simulink model "sampleModel2045_3_sub_sub"  (R2023a)
settings: Solver=VariableStepAuto  StartTime=0.0  StopTime=10.0  RelTol=1e-3
libraries: hdlsllib x5, simulink x2
settings Model: Creator=user1  LastModifiedBy=user1
settings OptimizationCC: BlockReduction=off  ConditionallyExecuteInputs=off

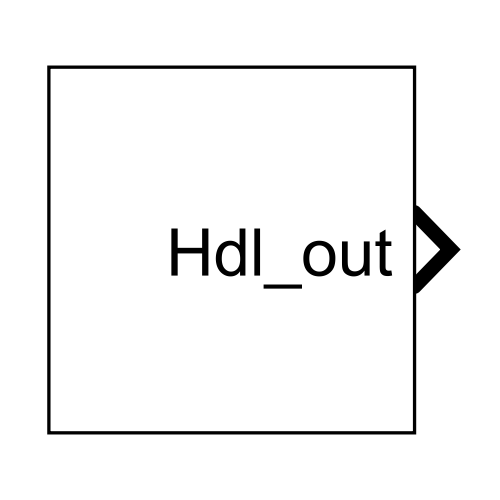
[thumbnail: Simulink's stored preview of the top-level diagram]
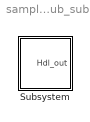
== system sampleModel2045_3_sub_sub ==
  Subsystem : Subsystem

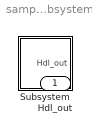
== system sampleModel2045_3_sub_sub/Subsystem ==
  Subsystem : Subsystem
  Hdl_out : Outport  OutDataTypeStr=uint8

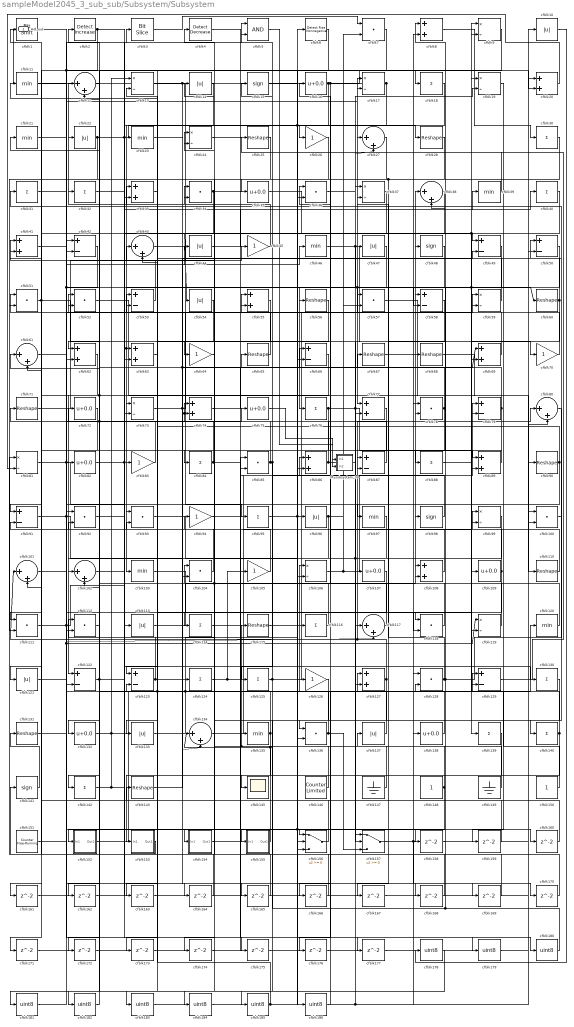
== system sampleModel2045_3_sub_sub/Subsystem/Subsystem ==
  Mysubsystem_34 : Subsystem  TreatAsAtomicUnit=on  RTWFcnName=Mysubsystem_34
      settings: RTWFcnNameOpts=User specified  RTWFileNameOpts=Use function name
  cfblk1 : hdlsllib/Logic and Bit Operations/Bit Shift  mode=Shift Left Logical  N=0
  cfblk{10,14,22,44,47,54,96,113,121,133,137} (11 alike) : Abs  OutDataTypeStr=uint8  SaturateOnIntegerOverflow=off
  cfblk{7,34,36,51..52,57,78,85,92..93,100,104,111..112,118,128,136} (17 alike) : DotProduct  OutDataTypeStr=uint8
  cfblk{12,27,38,43,61,80,101..102,117,134} (10 alike) : Sum  Inputs=|++  OutDataTypeStr=uint8
  cfblk{11,21,23,39,46,97,103,120,135} (9 alike) : MinMax  OutDataTypeStr=uint8
  cfblk{26,45,64,70,83,94,105,126} (8 alike) : Gain  OutDataTypeStr=uint8
  cfblk{9,13,17,19,24,37,59,73,81,99,106,119} (12 alike) : Product  Inputs=*/  OutDataTypeStr=uint8  RndMeth=Zero  SaturateOnIntegerOverflow=on
  cfblk{16,35,72,75,82,107,109,132,138} (9 alike) : Bias  Bias=0.0  SaturateOnIntegerOverflow=off
  cfblk{8,20,33,41,55,62..63,69,74,77,86,89,108,127} (14 alike) : Sum  OutDataTypeStr=uint8
  cfblk{25,28,56,60,65,67..68,71,90,110,115,131,143} (13 alike) : Reshape
  cfblk{18,30..32,40,76,84,88,95,114,116,124..125,130,139..140,142} (17 alike) : Sum  Inputs=+  OutDataTypeStr=uint8
  cfblk{42,49..50,53,58,66,79,87,91,122..123,129} (12 alike) : Sum  Inputs=+-  OutDataTypeStr=uint8
  cfblk{15,48,98,141} (4 alike) : Signum
  cfblk145 : Scope
  cfblk146 : hdlsllib/Sources/Counter Limited  uplimit=7  tsamp=-1
  cfblk147 : Ground
  cfblk148 : Constant  OutDataTypeStr=uint8  SampleTime=-1
  cfblk149 : Ground
  cfblk150 : Constant  OutDataTypeStr=uint8  SampleTime=-1
  cfblk151 : hdlsllib/Sources/Counter Free-Running  NumBits=16  tsamp=-1
  cfblk152 : Subsystem
      settings: LibrarySourceBlock=|
      | hdlsllib/Ports &
      | Subsystems/Subsystem
  cfblk153 : Subsystem
      settings: LibrarySourceBlock=|
      | hdlsllib/Ports &
      | Subsystems/Subsystem
  cfblk154 : Subsystem
      settings: LibrarySourceBlock=|
      | hdlsllib/Ports &
      | Subsystems/Subsystem
  cfblk155 : Subsystem
      settings: LibrarySourceBlock=|
      | hdlsllib/Ports &
      | Subsystems/Subsystem
  cfblk156 : Switch  OutDataTypeStr=uint8  SaturateOnIntegerOverflow=off  InputSameDT=off
  cfblk157 : Switch  OutDataTypeStr=uint8  SaturateOnIntegerOverflow=off  InputSameDT=off
  cfblk{158..177} (20 alike) : Delay  SampleTime=1
  cfblk{178..186} (9 alike) : DataTypeConversion  OutDataTypeStr=uint8  SaturateOnIntegerOverflow=off  RndMeth=Floor
  cfblk2 : simulink/Logic and Bit Operations/Detect Increase  vinit=0.0  OutDataTypeStr=uint8
      settings: LibrarySourceBlock=|
      | hdlsllib/Logic and Bit
      | Operations/Detect
      | Increase
  cfblk3 : hdlsllib/Logic and Bit Operations/Bit Slice  lidx=7  ridx=0
  cfblk4 : simulink/Logic and Bit Operations/Detect Decrease  vinit=0.0  OutDataTypeStr=uint8
      settings: LibrarySourceBlock=|
      | hdlsllib/Logic and Bit
      | Operations/Detect
      | Decrease
  cfblk5 : Logic  AllPortsSameDT=off  OutDataTypeStr=boolean
  cfblk6 : hdlsllib/Logic and Bit Operations/Detect Rise Nonnegative  vinit=0  OutDataTypeStr=uint8
  Hdl_out : Outport  OutDataTypeStr=uint8
  wires:
  cfblk75/1 -> Mysubsystem_34/2(In2)
  cfblk5/1 -> Mysubsystem_34/1(In1)
  cfblk186/1 -> cfblk126/1
  cfblk15/1 -> cfblk186/1
  cfblk185/1 -> cfblk143/1, cfblk100/1
  cfblk184/1 -> cfblk6/1
  cfblk38/1 -> cfblk184/1
  cfblk183/1 -> cfblk117/1, cfblk138/1
  cfblk182/1 -> cfblk92/2
  cfblk181/1 -> cfblk92/1
  cfblk178/1 -> cfblk181/1
  cfblk180/1 -> cfblk128/2, cfblk65/1
  cfblk179/1 -> cfblk10/1
  cfblk4/1 -> cfblk179/1
  cfblk10/1 -> cfblk178/1
  cfblk177/1 -> cfblk80/2
  cfblk32/1 -> cfblk177/1
  cfblk176/1 -> cfblk128/1
  cfblk139/1 -> cfblk176/1
  cfblk175/1 -> cfblk20/1
  cfblk31/1 -> cfblk175/1
  cfblk174/1 -> cfblk86/2
  cfblk130/1 -> cfblk174/1
  cfblk173/1 -> cfblk37/1
  cfblk107/1 -> cfblk173/1
  cfblk172/1 -> cfblk85/2
  cfblk171/1 -> cfblk77/2
  cfblk170/1 -> cfblk102/2
  cfblk169/1 -> cfblk91/2
  cfblk168/1 -> cfblk34/2
  cfblk167/1 -> cfblk78/1
  cfblk58/1 -> cfblk167/1
  cfblk166/1 -> cfblk81/1
  cfblk165/1 -> cfblk42/1
  cfblk164/1 -> cfblk123/2
  cfblk61/1 -> cfblk164/1
  cfblk163/1 -> cfblk50/2
  cfblk63/1 -> cfblk163/1
  cfblk162/1 -> cfblk8/2
  cfblk161/1 -> cfblk33/2
  cfblk160/1 -> cfblk38/2
  cfblk159/1 -> cfblk1/1
  cfblk19/1 -> cfblk159/1
  cfblk158/1 -> cfblk108/2
  cfblk24/1 -> cfblk158/1
  cfblk30/1 -> cfblk154/1(In1)
  cfblk102/1 -> cfblk44/1
  cfblk25/1 -> cfblk35/1
  cfblk78/1 -> cfblk22/1, cfblk121/1
  cfblk9/1 -> cfblk36/2
  cfblk91/1 -> cfblk124/1, cfblk118/2
  cfblk69/1 -> cfblk55/1
  cfblk119/1 -> cfblk37/2
  cfblk85/1 -> cfblk125/1, cfblk55/2, cfblk53/2
  cfblk27/1 -> cfblk51/2
  cfblk54/1 -> cfblk64/1
  cfblk17/1 -> cfblk66/2, cfblk63/2, Hdl_out/1
  cfblk74/1 -> cfblk67/1
  cfblk1/1 -> cfblk156/1, cfblk60/1, cfblk20/2
  cfblk147/1 -> cfblk112/1
  cfblk23/1 -> cfblk157/2, cfblk156/3
  cfblk2/1 -> cfblk101/2, cfblk130/1
  cfblk50/1 -> cfblk88/1, cfblk119/2
  cfblk92/1 -> cfblk180/1
  cfblk66/1 -> cfblk161/1, cfblk162/1
  cfblk37/1 -> cfblk133/1
  cfblk28/1 -> cfblk42/2, cfblk97/1
  cfblk132/1 -> cfblk120/1, cfblk23/1
  cfblk72/1 -> cfblk111/1
  cfblk60/1 -> cfblk36/1, cfblk99/2
  cfblk11/1 -> cfblk56/1
  cfblk86/1 -> cfblk47/1, cfblk14/1
  cfblk76/1 -> cfblk89/1, cfblk27/2, cfblk84/1
  cfblk127/1 -> cfblk101/1, cfblk107/1, cfblk136/2
  cfblk143/1 -> cfblk66/1
  cfblk136/1 -> cfblk2/1, cfblk13/2, cfblk157/3
  cfblk51/1 -> cfblk157/1, cfblk171/1
  cfblk153/1(Out1) -> cfblk141/1
  cfblk151/1 -> cfblk127/1
  cfblk47/1 -> cfblk77/1, cfblk156/2
  cfblk133/1 -> cfblk106/2, cfblk9/2
  cfblk7/1 -> cfblk152/1(In1)
  cfblk101/1 -> cfblk3/1
  cfblk118/1 -> cfblk51/1
  cfblk12/1 -> cfblk82/1
  cfblk42/1 -> cfblk62/2
  cfblk3/1 -> cfblk7/1
  cfblk111/1 -> cfblk73/2, cfblk57/1
  cfblk83/1 -> cfblk41/2, cfblk32/1
  cfblk35/1 -> cfblk109/1
  cfblk140/1 -> cfblk153/1(In1), cfblk68/1
  cfblk90/1 -> cfblk33/1, cfblk112/2
  cfblk41/1 -> cfblk17/2
  cfblk39/1 -> cfblk27/1
  cfblk154/1(Out1) -> cfblk108/1
  cfblk121/1 -> cfblk75/1
  cfblk36/1 -> cfblk19/2
  cfblk98/1 -> cfblk15/1
  cfblk6/1 -> cfblk183/1
  cfblk155/1(Out1) -> cfblk93/2, cfblk134/1
  cfblk131/1 -> cfblk46/1, cfblk119/1
  cfblk84/1 -> cfblk52/1, cfblk118/1
  cfblk88/1 -> cfblk19/1
  cfblk82/1 -> cfblk5/1, cfblk104/2
  cfblk57/1 -> cfblk79/2
  cfblk94/1 -> cfblk87/2
  cfblk64/1 -> cfblk34/1
  cfblk73/1 -> cfblk69/1, cfblk49/2, cfblk17/1, cfblk134/2
  cfblk48/1 -> cfblk76/1
  cfblk103/1 -> cfblk129/2
  cfblk55/1 -> cfblk114/1
  cfblk34/1 -> cfblk91/1, cfblk69/2
  cfblk81/1 -> cfblk113/1, cfblk117/2
  cfblk67/1 -> cfblk100/2
  cfblk152/1(Out1) -> cfblk96/1
  cfblk8/1 -> cfblk30/1
  cfblk26/1 -> cfblk62/1
  cfblk97/1 -> cfblk132/1, cfblk127/2
  cfblk105/1 -> cfblk4/1
  cfblk93/1 -> cfblk116/1
  cfblk68/1 -> cfblk110/1
  cfblk112/1 -> cfblk12/2
  cfblk150/1 -> cfblk129/1
  cfblk99/1 -> cfblk142/1
  cfblk77/1 -> cfblk102/1
  cfblk65/1 -> cfblk24/2
  cfblk124/1 -> cfblk85/1, cfblk105/1
  cfblk22/1 -> cfblk28/1, cfblk49/1, cfblk111/2
  cfblk106/1 -> cfblk78/2, cfblk7/2
  cfblk70/1 -> cfblk8/1
  cfblk87/1 -> cfblk71/1
  cfblk44/1 -> cfblk40/1
  cfblk18/1 -> cfblk43/2
  cfblk156/1 -> cfblk135/1
  cfblk138/1 -> cfblk24/1
  cfblk52/1 -> cfblk139/1
  cfblk157/1 -> cfblk90/1, cfblk170/1
  cfblk148/1 -> cfblk43/1, cfblk182/1
  cfblk116/1 -> cfblk104/1
  cfblk100/1 -> cfblk50/1
  cfblk16/1 -> cfblk18/1, cfblk136/1, cfblk26/1
  cfblk46/1 -> cfblk70/1, cfblk58/2
  cfblk122/1 -> cfblk39/1, cfblk172/1
  cfblk21/1 -> cfblk122/2
  cfblk142/1 -> cfblk13/1, cfblk165/1
  cfblk89/1 -> cfblk83/1
  cfblk59/1 -> cfblk11/1
  cfblk80/1 -> cfblk140/1
  cfblk62/1 -> cfblk122/1
  cfblk125/1 -> cfblk98/1, cfblk5/2
  cfblk43/1 -> cfblk59/2
  cfblk40/1 -> cfblk54/1, cfblk89/2
  cfblk146/1 -> cfblk74/1, cfblk74/2, cfblk115/1
  cfblk95/1 -> cfblk79/1, cfblk168/1
  cfblk123/1 -> cfblk72/1, cfblk160/1
  cfblk20/1 -> cfblk81/2
  cfblk56/1 -> cfblk93/1
  cfblk71/1 -> cfblk45/1
  cfblk110/1 -> cfblk16/1
  cfblk114/1 -> cfblk9/1
  cfblk53/1 -> cfblk41/1
  cfblk13/1 -> cfblk95/1, cfblk169/1
  cfblk134/1 -> cfblk87/1
  cfblk120/1 -> cfblk21/1, cfblk94/1
  cfblk117/1 -> cfblk86/1
  cfblk108/1 -> cfblk38/1
  cfblk129/1 -> cfblk25/1
  cfblk33/1 -> cfblk123/1
  cfblk137/1 -> cfblk106/1
  cfblk104/1 -> cfblk61/2
  cfblk141/1 -> cfblk131/1
  cfblk135/1 -> cfblk145/1, cfblk53/1
  cfblk79/1 -> cfblk58/1, cfblk166/1
  cfblk115/1 -> cfblk59/1
  cfblk45/1 -> cfblk12/1
  cfblk14/1 -> cfblk73/1
  cfblk128/1 -> cfblk31/1, cfblk48/1, cfblk52/2
  cfblk113/1 -> cfblk80/1
  cfblk96/1 -> cfblk61/1, cfblk57/2
  cfblk49/1 -> cfblk103/1, cfblk63/1
  cfblk149/1 -> cfblk137/1
  cfblk109/1 -> cfblk155/1(In1), cfblk99/1
  cfblk126/1 -> cfblk185/1

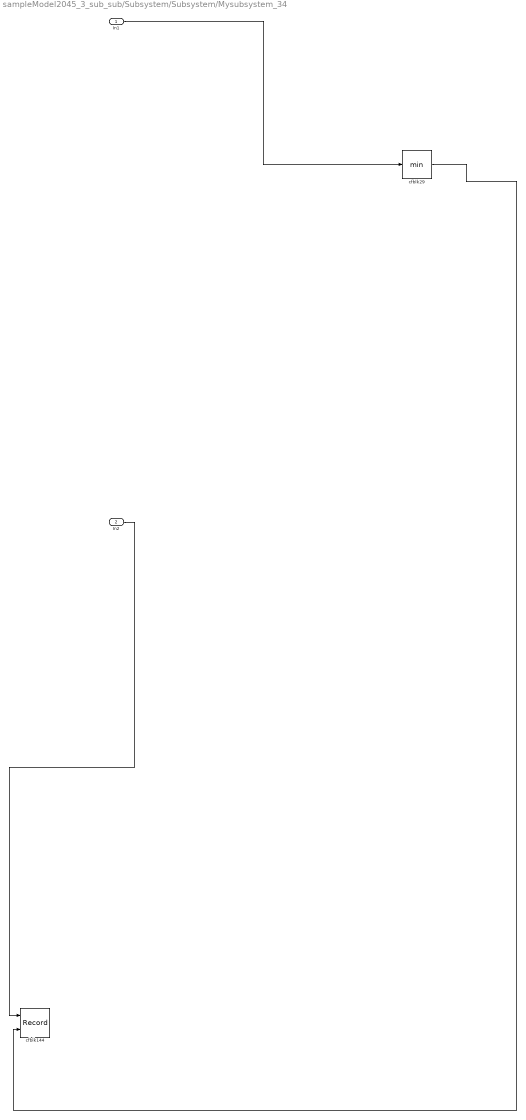
== system sampleModel2045_3_sub_sub/Subsystem/Subsystem/Mysubsystem_34 ==
  In1 : Inport
  In2 : Inport  Port=2
  cfblk144 : Record  FileSettingsInternal="{\"entries\":[{\"content\":{\"excelSettings\":{\"content\":{},\"type\":\"Streamout.ExcelSettings\"}},\"type\":\"Streamout.FileSettingStorage\",\"uuid\":\"\"}],\"packageUris\":[\"http:\\/\\/schema.mathworks.com\\/mf0\\/streamout_blocks\\/R2020a\"],\"version\":\"1.0\"}"  Layout=[1 1]  SignalsInternal="{\"entries\":[{\"content\":{},\"type\":\"RecordBlkView.InputSignals\",\"uuid\":\"\"}],\"packageUris\":[\"http:\\/\\/schema.mathworks.com\\/mf0\\/streamout_blocks\\/R2020a\"],\"version\":\"1.0\"}"  VisualizationBindings="{\"xyplotplugin\":{\"info\":[{\"series\":[],\"subplotID\":1}]}}"  CompatibilityTag=XY  st=-1
  cfblk29 : MinMax
  wires:
  In2/1 -> cfblk144/1
  cfblk29/1 -> cfblk144/2
  In1/1 -> cfblk29/1

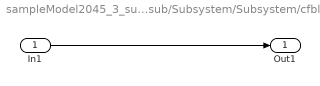
== system sampleModel2045_3_sub_sub/Subsystem/Subsystem/cfblk152 ==
  In1 : Inport
  Out1 : Outport
  wires:
  In1/1 -> Out1/1

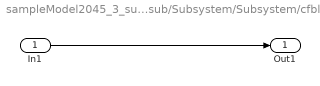
== system sampleModel2045_3_sub_sub/Subsystem/Subsystem/cfblk153 ==
  In1 : Inport
  Out1 : Outport
  wires:
  In1/1 -> Out1/1

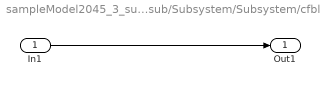
== system sampleModel2045_3_sub_sub/Subsystem/Subsystem/cfblk154 ==
  In1 : Inport
  Out1 : Outport
  wires:
  In1/1 -> Out1/1

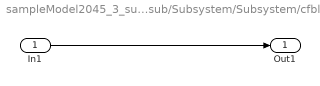
== system sampleModel2045_3_sub_sub/Subsystem/Subsystem/cfblk155 ==
  In1 : Inport
  Out1 : Outport
  wires:
  In1/1 -> Out1/1
